simulink model "sim_4_twolink_impedance_control"  (R2021a)
settings: Solver=VariableStepAuto  StartTime=0.0  StopTime=12  MaxStep=0.01  RelTol=1e-3
values from neighbouring files (symbols this model uses):
  b1 = 0.01    [sim_params.m]    (also in sim_params_force.m)
  b2 = 0.01    [sim_params.m]    (also in sim_params_force.m)
  D = [zeros(n); eye(n)]    [control_comparison_script.m]    (also in gen_twolink_ss.m = reshape([0.0,0.0,0.0,0.0,0.0,0.0,0.0,0.0],[4,2]))
  g = 9.80665    [sim_params.m]    (also in sim_params_force.m)
  L1x = 0.3    [sim_params.m]    (also in sim_params_force.m)
  L1y = 0.050    (= 0.05)    [sim_params.m]    (also in sim_params_force.m)
  L1z = 0.05    [sim_params.m]    (also in sim_params_force.m)
  L2x = 0.15    [sim_params.m]    (also in sim_params_force.m = 0.3)
  L2y = 0.05    [sim_params.m]    (also in sim_params_force.m)
  L2z = 0.05    [sim_params.m]    (also in sim_params_force.m)
  m1 = m1*1.25    [control_comparison_script.m]    (also in sim_params.m = 2.775; sim_params_force.m = 2.775)
  m2 = m2*1.25    [control_comparison_script.m]    (also in sim_params.m = 1.3875; sim_params_force.m = 2.775)
  max_joint_torque1 = 20    [sim_params.m]    (also in sim_params_force.m)
  max_joint_torque2 = 10    [sim_params.m]    (also in sim_params_force.m = 20)
  theta1_0 = 0    [sim_params.m]    (also in sim_params_force.m = 1.57079632679)
  theta1_dot_0 = 0    [sim_params.m]    (also in sim_params_force.m)
  theta2_0 = 0    [sim_params.m]    (also in sim_params_force.m = -1.57079632679)
  theta2_dot_0 = 0    [sim_params.m]    (also in sim_params_force.m)
undefined symbols (not defined in the file or in its folder): FT_control, Impedance_no, Kdt, Ke_d, Ke_s, Kpt, Levenberg, Marquardt, Mt_inv, R_env, sigbuilder_block, W_env, X, Xenv, Y, Z
libraries: sm_lib x77, nesl_utility x58, pid_lib x6, simulink x6, robotmaniplib x3, robotcorelib x1
(part 1 of 5)
settings Model: Creator=Petronas-Tareq  LastModifiedBy=Petronas-Tareq
settings ExplorerConfigSet: InternalSimMechanicsExplorerSettings="<ExplorerConfiguration><canonicalview>default</canonicalview><AnimationSetting><BasePlaybackSpeed>1.0</BasePlaybackSpeed><PlaybackSpeedFactor>1.0</PlaybackSpeedFactor></AnimationSetting><TilePanel><TileInfo><Tiles Columns=\"2\" Count=\"4\" Rows=\"2\"><Column Weight=\"0.4998\"/><Column Weight=\"0.5002\"/><Row Weight=\"0.5\"/><Row Weight=\"0.5\"/><Tile Height=\"1\" Width=\"1\" X=\"0\" Y=\"0\"/><Tile Height=\"1\" Width=\"1\" X=\"0\" Y=\"1\"/><Tile Height=\"1\" Width=\"1\" X=\"1\" Y=\"0\"/><Tile Height=\"1\" Width=\"1\" X=\"1\" Y=\"1\"/></Tiles></TileInfo><SceneInfo><SceneViewer><BGColor><R>0.60000002384185791</R><G>0.60000002384185791</G><B>0.60000002384185791</B></BGColor><Camera><DoPerspective>off</DoPerspective><Position><X>0.22866161329300444</X><Y>-0.999999955971509147</Y><Z>-4.12820655437684536e-09</Z></Position><Center><X>0.22866161329300444</X><Y>4.40284908531651742e-08</Y><Z>-4.12820655437684536e-09</Z></Center><Up><X>0</X><Y>-0</Y><Z>1</Z></Up><ViewLimDist>1</ViewLimDist><YLim>0.257500000000000007</YLim><XLim>0.552253577106518345</XLim></Camera></SceneViewer><SceneViewer><BGColor><R>0.60000002384185791</R><G>0.60000002384185791</G><B>0.60000002384185791</B></BGColor><Camera><DoPerspective>off</DoPerspective><Position><X>0.204072367525804987</X><Y>-2.34335064047906805</Y><Z>0.167988192192854713</Z></Position><Center><X>0.219660802383778442</X><Y>-1.34642671678176962</Y><Z>0.0911787457755401237</Z></Center><Up><X>-0.0262288638413234881</X><Y>0.0772000539040926803</Y><Z>0.996670556592697987</Z></Up><ViewLimDist>1</ViewLimDist><YLim>0.515000000000000013</YLim><XLim>1.10450715421303669</XLim></Camera></SceneViewer><SceneViewer><BGColor><R>0.60000002384185791</R><G>0.60000002384185791</G><B>0.60000002384185791</B></BGColor><Camera><DoPerspective>off</DoPerspective><Position><X>-0.24899486320315789</X><Y>-0.765272772333560392</Y><Z>0.697835060620221048</Z></Position><Center><X>0.26973731486207464</X><Y>-0.211131790133127217</Y><Z>0.0468014982858467876</Z></Center><Up><X>0.244353234025975474</X><Y>0.633635300715601257</Y><Z>0.734028475406845016</Z></Up><ViewLimDist>1</ViewLimDist><YLim>0.431008132994174953</YLim><XLim>0.925057201179866673</XLim></Camera></SceneViewer><SceneViewer><BGColor><R>0.60000002384185791</R><G>0.60000002384185791</G><B>0.60000002384185791</B></BGColor><Camera><DoPerspective>off</DoPerspective><Position><X>0.236408339938699752</X><Y>-3.48082895840207129e-09</Y><Z>0.999999999307370047</Z></Position><Center><X>0.236408339938699752</X><Y>-3.48082895840207129e-09</Y><Z>-6.9262995339158806e-10</Z></Center><Up><X>0</X><Y>1</Y><Z>-0</Z></Up><ViewLimDist>1</ViewLimDist><YLim>0.515000000000000013</YLim><XLim>1.10532591414944359</XLim></Camera></SceneViewer></SceneInfo></TilePanel><MechEditorPanel><Cameras/><GfxPanelCameraMap/><VideoCreator><PlaybackSpeedRatio>1.0</PlaybackSpeedRatio><FrameRate>30</FrameRate><VideoFormat>Motion JPEG AVI</VideoFormat><FrameSize>auto</FrameSize></VideoCreator></MechEditorPanel></ExplorerConfiguration>"

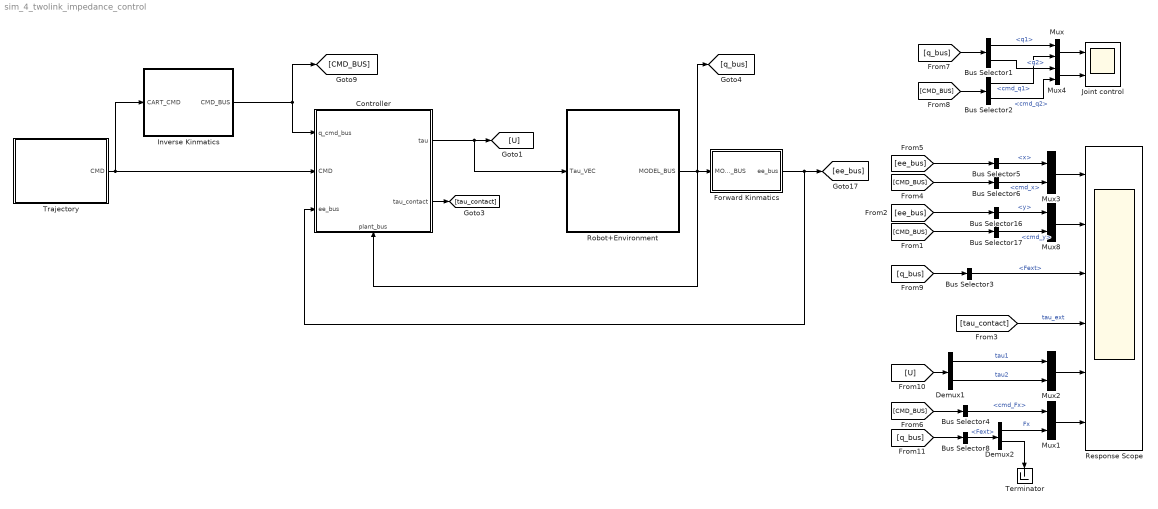
== system sim_4_twolink_impedance_control ==
  Bus Selector1 : BusSelector  OutputSignals=q1,q2
  Bus Selector16 : BusSelector  OutputSignals=y
  Bus Selector17 : BusSelector  OutputSignals=cmd_y
  Bus Selector2 : BusSelector  OutputSignals=cmd_q1,cmd_q2
  Bus Selector3 : BusSelector  OutputSignals=Fext
  Bus Selector4 : BusSelector  OutputSignals=cmd_Fx
  Bus Selector5 : BusSelector  OutputSignals=x
  Bus Selector6 : BusSelector  OutputSignals=cmd_x
  Bus Selector8 : BusSelector  OutputSignals=Fext
  Controller : Subsystem  Variant=on  VariantControlMode=label  LabelModeActiveChoice=Impedance_FT_control  PropagateVariantConditions=on
      settings: PortSchema="{\"entries\":[{\"content\":{\"sides\":[{\"content\":{\"connectorIds\":[\"In1\",\"In2\",\"In3\"]},\"type\":\"ConnectorPlacement.EquallySpacedRectSide\",\"uuid\":\"12e0e0c2-14f8-4f2c-9d40-c223a4f2431c\"},{\"content\":{\"connectorIds\":[\"Out1\",\"Out2\"],\"side\":\"RIGHT\"},\"type\":\"ConnectorPlacement.EquallySpacedRectSide\",\"uuid\":\"b8197539-8519-4525-8d0f-ad401569c0d0\"},{\"content\":{\"connectorIds\":[],\"side\":\"TOP\"},\"type\":\"ConnectorPlacement.EquallySpacedRectSide\",\"uuid\":\"f43dc380-71af-4005-ac59-0dbedf3cc41e\"},{\"content\":{\"connectorIds\":[\"In4\"],\"side\":\"BOTTOM\"},\"type\":\"ConnectorPlacement.EquallySpacedRectSide\",\"uuid\":\"0d04f827-4285-4524-8874-ff3126ed5eeb\"}]},\"type\":\"ConnectorPlacement.EquallySpacedConnector\",\"uuid\":\"aec7d64b-efe7-424b-994a-6b7ee567ecbd\"}],\"packageUris\":[\"http://schema.mathworks.com/mf0/Connector/R2020b\"],\"version\":\"1.0\"}"
  Demux1 : Demux  Outputs=2
  Demux2 : Demux  Outputs=2
  Forward Kinmatics : Subsystem
  Inverse Kinmatics : Subsystem
  Joint control : Scope  NumInputPorts=2
  Mux{,1..4,8} (6 alike) : Mux  Inputs=2
  Response Scope : Scope  NumInputPorts=6
  Robot+Environment : Subsystem  Variant=on  VariantControlMode=label  LabelModeActiveChoice=Choice1
  Terminator : Terminator
  Trajectory : Subsystem  Variant=on  VariantControlMode=label  LabelModeActiveChoice=ramp
  wires:
  Trajectory/1(CMD) -> Inverse Kinmatics/1(CART_CMD), Controller/2(CMD)
  Controller/1(tau) -> [U], Robot+Environment/1(Tau_VEC)
  Robot+Environment/1(MODEL_BUS) -> Controller/4(plant_bus), Forward Kinmatics/1(MODEL_BUS), [q_bus]
  Bus Selector2/1 -> Mux/2  "<cmd_q1>"
  Bus Selector1/2 -> Mux4/1  "<q2>"
  Mux4/1 -> Joint control/2
  [CMD_BUS] -> Bus Selector2/1
  Bus Selector1/1 -> Mux/1  "<q1>"
  Mux/1 -> Joint control/1
  Bus Selector2/2 -> Mux4/2  "<cmd_q2>"
  [q_bus] -> Bus Selector1/1
  Inverse Kinmatics/1(CMD_BUS) -> Controller/1(q_cmd_bus), [CMD_BUS]
  [ee_bus] -> Bus Selector5/1
  [tau_contact] -> Response Scope/4  "tau_ext"
  Bus Selector17/1 -> Mux8/2  "<cmd_y>"
  Mux2/1 -> Response Scope/5
  [U] -> Demux1/1
  [CMD_BUS] -> Bus Selector17/1
  Bus Selector16/1 -> Mux8/1  "<y>"
  Demux1/2 -> Mux2/2  "tau2"
  [ee_bus] -> Bus Selector16/1
  Demux1/1 -> Mux2/1  "tau1"
  Mux8/1 -> Response Scope/2
  Bus Selector6/1 -> Mux3/2  "<cmd_x>"
  [CMD_BUS] -> Bus Selector6/1
  Bus Selector5/1 -> Mux3/1  "<x>"
  Mux3/1 -> Response Scope/1
  Forward Kinmatics/1(ee_bus) -> Controller/3(ee_bus), [ee_bus]
  [q_bus] -> Bus Selector3/1
  Bus Selector3/1 -> Response Scope/3  "<Fext>"
  Controller/2(tau_contact) -> [tau_contact]
  Mux1/1 -> Response Scope/6
  [CMD_BUS] -> Bus Selector4/1
  Bus Selector4/1 -> Mux1/1  "<cmd_Fx>"
  [q_bus] -> Bus Selector8/1
  Bus Selector8/1 -> Demux2/1  "<Fext>"
  Demux2/1 -> Mux1/2  "Fx"
  Demux2/2 -> Terminator/1

== system sim_4_twolink_impedance_control/Controller ==
  note: 1) Add Subsystem or Model blocks as valid variant choices.
      | 2) You cannot connect blocks at this level. At simulation, connectivity is automatically
      | determined, based on the active variant and port name matching.
  q_cmd_bus : Inport
  CMD : Inport  Port=2
  ee_bus : Inport  Port=3
  plant_bus : Inport  Port=4
  "Impedance (with F/T) +Inverse Dynamics control " : Subsystem  VariantControl=Impedance_FT_control
  "Impedance (without F/T) + Inverse Dynamics control " : Subsystem  VariantControl=Impedance_no/FT_control
  Simple complaince Control : Subsystem  VariantControl=simple_complaince_control
  tau : Outport
  tau_contact : Outport  Port=2

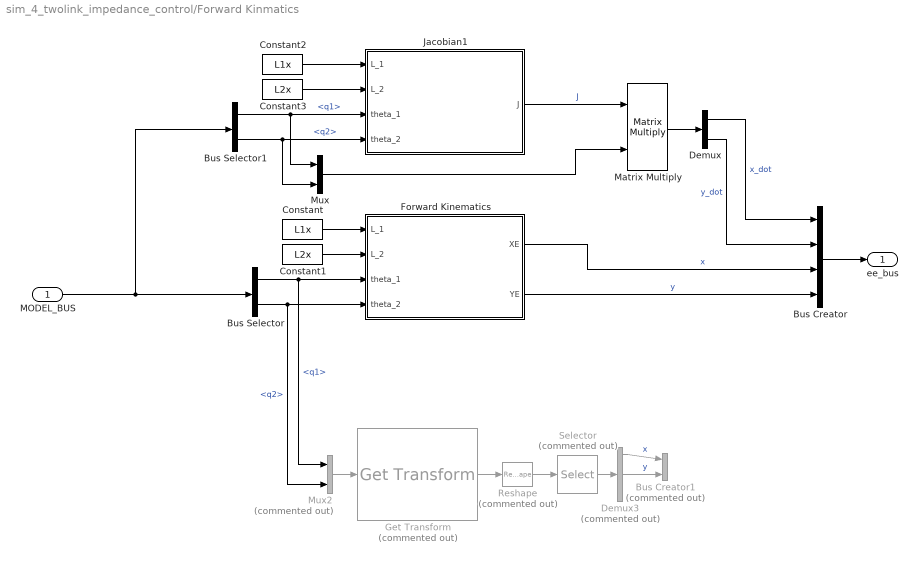
== system sim_4_twolink_impedance_control/Forward Kinmatics ==
  MODEL_BUS : Inport
  Bus Creator : BusCreator  Inputs=4
  Bus Creator1 : BusCreator  Commented=on  Inputs=2
  Bus Selector : BusSelector  OutputSignals=q1,q2
  Bus Selector1 : BusSelector  OutputSignals=q1,q2
  Constant : Constant  Value=L1x
  Constant1 : Constant  Value=L2x
  Constant2 : Constant  Value=L1x
  Constant3 : Constant  Value=L2x
  Demux : Demux  Outputs=2
  Demux3 : Demux  Commented=on  Outputs=3
  Forward Kinematics : MATLAB Function  TreatAsAtomicUnit=on
  Get Transform : robotmaniplib/Get Transform  Commented=on  RigidBodyTree=RR_robot  SourceBody=end_effector  TargetBody=base  SimulateUsing=Interpreted execution
  Jacobian1 : MATLAB Function  TreatAsAtomicUnit=on
  Matrix Multiply : Product  Multiplication=Matrix(*)
  Mux : Mux  Inputs=2
  Mux2 : Mux  Commented=on  Inputs=2
  Reshape : Reshape  Commented=on
  Selector : Selector  Commented=on  InputPortWidth=16  IndexOptions=Index vector (dialog)  Indices=[13:15]  OutputSizes=1
  ee_bus : Outport
  wires:
  Forward Kinematics/2(YE) -> Bus Creator/4  "y"
  Forward Kinematics/1(XE) -> Bus Creator/3  "x"
  Bus Selector/1 -> Mux2/1, Forward Kinematics/3(theta_1)  "<q1>"
  Bus Selector/2 -> Mux2/2, Forward Kinematics/4(theta_2)  "<q2>"
  Constant/1 -> Forward Kinematics/1(L_1)
  Constant1/1 -> Forward Kinematics/2(L_2)
  Mux2/1 -> Get Transform/1
  Get Transform/1 -> Reshape/1
  Reshape/1 -> Selector/1
  Selector/1 -> Demux3/1
  Demux3/1 -> Bus Creator1/1  "x"
  Demux3/2 -> Bus Creator1/2  "y"
  Bus Creator/1 -> ee_bus/1
  Constant2/1 -> Jacobian1/1(L_1)
  Constant3/1 -> Jacobian1/2(L_2)
  Jacobian1/1(J) -> Matrix Multiply/1  "J"
  Bus Selector1/2 -> Mux/2, Jacobian1/4(theta_2)  "<q2>"
  MODEL_BUS/1 -> Bus Selector1/1, Bus Selector/1
  Bus Selector1/1 -> Mux/1, Jacobian1/3(theta_1)  "<q1>"
  Mux/1 -> Matrix Multiply/2
  Matrix Multiply/1 -> Demux/1
  Demux/1 -> Bus Creator/1  "x_dot"
  Demux/2 -> Bus Creator/2  "y_dot"

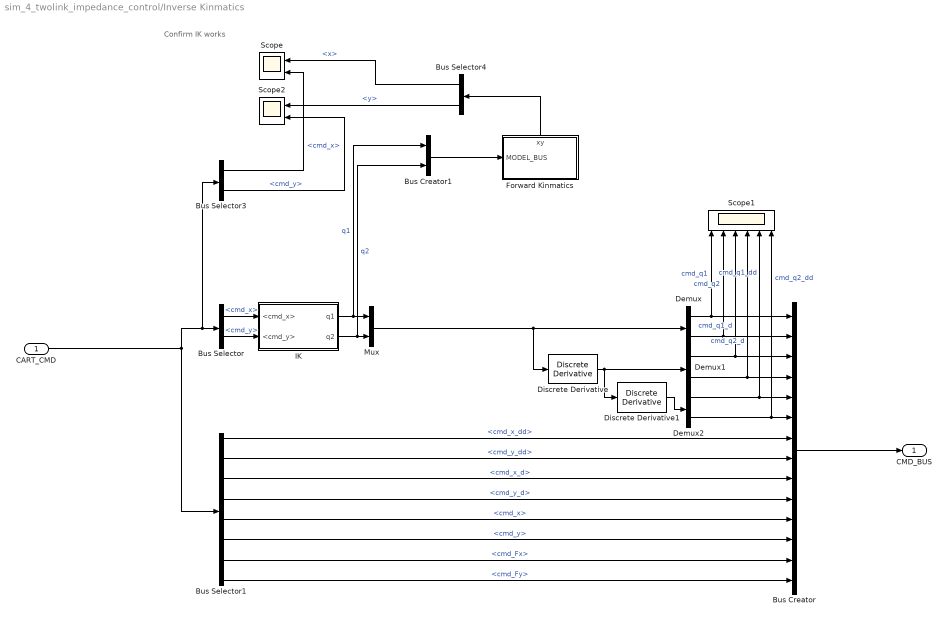
== system sim_4_twolink_impedance_control/Inverse Kinmatics ==
  note: Confirm IK works
  CART_CMD : Inport
  Bus Creator : BusCreator  Inputs=14
  Bus Creator1 : BusCreator  Inputs=2
  Bus Selector : BusSelector  OutputSignals=cmd_x,cmd_y
  Bus Selector1 : BusSelector  OutputSignals=cmd_x_dd,cmd_y_dd,cmd_x_d,cmd_y_d,cmd_x,cmd_y,cmd_Fx,cmd_Fy
  Bus Selector3 : BusSelector  OutputSignals=cmd_x,cmd_y
  Bus Selector4 : BusSelector  OutputSignals=x,y
  Demux : Demux  Outputs=2
  Demux1 : Demux  Outputs=2
  Demux2 : Demux  Outputs=2
  Discrete Derivative : simulink/Discrete/Discrete Derivative  gainval=1.0  ICPrevScaledInput=0.0  OutMin=[]  OutMax=[]  OutDataType=fixdt(1, 16)  OutScaling=2^-10  DoSatur=off
  Discrete Derivative1 : simulink/Discrete/Discrete Derivative  gainval=1.0  ICPrevScaledInput=0.0  OutMin=[]  OutMax=[]  OutDataType=fixdt(1, 16)  OutScaling=2^-10  DoSatur=off
  Forward Kinmatics : Subsystem
      settings: PortSchema="{\"entries\":[{\"content\":{\"sides\":[{\"content\":{\"connectorIds\":[\"In1\"]},\"type\":\"ConnectorPlacement.EquallySpacedRectSide\",\"uuid\":\"2c0f0405-b445-4922-82b0-9ed34ea6e343\"},{\"content\":{\"connectorIds\":[],\"side\":\"RIGHT\"},\"type\":\"ConnectorPlacement.EquallySpacedRectSide\",\"uuid\":\"91fea7c3-4850-470e-b524-5886f9b138cb\"},{\"content\":{\"connectorIds\":[\"Out1\"],\"side\":\"TOP\"},\"type\":\"ConnectorPlacement.EquallySpacedRectSide\",\"uuid\":\"51029b8b-093e-4a55-82a5-f93421c28d2e\"}]},\"type\":\"ConnectorPlacement.EquallySpacedConnector\",\"uuid\":\"843aee16-b8cd-4273-ac03-a5f22ed539be\"}],\"packageUris\":[\"http://schema.mathworks.com/mf0/Connector/R2020b\"],\"version\":\"1.0\"}"
  IK : Subsystem
  Mux : Mux  Inputs=2
  Scope : Scope  NumInputPorts=2
  Scope1 : Scope  NumInputPorts=6
  Scope2 : Scope  NumInputPorts=2
  CMD_BUS : Outport
  wires:
  CART_CMD/1 -> Bus Selector3/1, Bus Selector/1, Bus Selector1/1
  Bus Selector1/1 -> Bus Creator/7  "<cmd_x_dd>"
  Bus Selector1/2 -> Bus Creator/8  "<cmd_y_dd>"
  Bus Selector1/3 -> Bus Creator/9  "<cmd_x_d>"
  Bus Selector1/4 -> Bus Creator/10  "<cmd_y_d>"
  Bus Selector1/5 -> Bus Creator/11  "<cmd_x>"
  Bus Selector1/6 -> Bus Creator/12  "<cmd_y>"
  Demux1/1 -> Scope1/3, Bus Creator/3  "cmd_q1_d"
  Demux2/2 -> Scope1/6, Bus Creator/6  "cmd_q2_dd"
  Demux1/2 -> Scope1/4, Bus Creator/4  "cmd_q2_d"
  Demux/1 -> Scope1/1, Bus Creator/1  "cmd_q1"
  Demux/2 -> Scope1/2, Bus Creator/2  "cmd_q2"
  Bus Selector/1 -> IK/1(<cmd_x>)  "<cmd_x>"
  Bus Selector/2 -> IK/2(<cmd_y>)  "<cmd_y>"
  IK/1(q1) -> Bus Creator1/1, Mux/1  "q1"
  IK/2(q2) -> Bus Creator1/2, Mux/2  "q2"
  Mux/1 -> Demux/1, Discrete Derivative/1
  Discrete Derivative/1 -> Demux1/1, Discrete Derivative1/1
  Demux2/1 -> Scope1/5, Bus Creator/5  "cmd_q1_dd"
  Discrete Derivative1/1 -> Demux2/1
  Bus Creator/1 -> CMD_BUS/1
  Bus Creator1/1 -> Forward Kinmatics/1(MODEL_BUS)
  Forward Kinmatics/1(xy) -> Bus Selector4/1
  Bus Selector3/1 -> Scope/2  "<cmd_x>"
  Bus Selector4/1 -> Scope/1  "<x>"
  Bus Selector4/2 -> Scope2/1  "<y>"
  Bus Selector3/2 -> Scope2/2  "<cmd_y>"
  Bus Selector1/7 -> Bus Creator/13  "<cmd_Fx>"
  Bus Selector1/8 -> Bus Creator/14  "<cmd_Fy>"

== system sim_4_twolink_impedance_control/Robot+Environment ==
  note: 1) Add Subsystem or Model blocks as valid variant choices.
      | 2) You cannot connect blocks at this level. At simulation, connectivity is automatically
      | determined, based on the active variant and port name matching.
  Tau_VEC : Inport
  ARM+Wall Simscape : Subsystem  VariantControl=Choice1
  ARM+Wall Simulink : Subsystem  VariantControl=Choice2
  ARM+curve Simscape : Subsystem  VariantControl=Choice3
  ARM+extrude Simscape : Subsystem  VariantControl=Choice4
  ARM+no constraints Simscape : Subsystem  VariantControl=Choice5
  ARM+ramp up Simscape : Subsystem  VariantControl=Choice6
  MODEL_BUS : Outport

== system sim_4_twolink_impedance_control/Trajectory ==
  note: 1) Add Subsystem or Model blocks as valid variant choices.
      | 2) You cannot connect blocks at this level. At simulation, connectivity is automatically
      | determined, based on the active variant and port name matching.
  Step command : Subsystem  VariantControl=step
  ramp command : Subsystem  VariantControl=ramp
  CMD : Outport

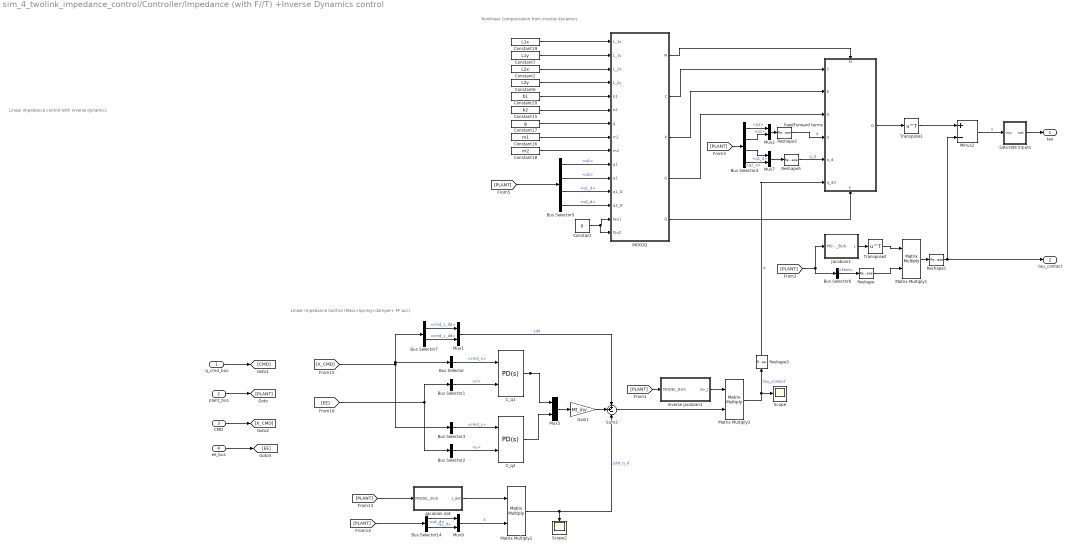
== system sim_4_twolink_impedance_control/Controller/Impedance (with F//T) +Inverse Dynamics control  ==
  note: Linear impedance control with inverse dynamics
  note: Nonlinear Compensation from inverse dynamics
  note: Linear Impedance Control (Mass+Spring+damper+ FF acc)
  q_cmd_bus : Inport
  plant_bus : Inport  Port=2
  CMD : Inport  Port=3
  ee_bus : Inport  Port=4
  Bus Selector : BusSelector  OutputSignals=cmd_x
  Bus Selector1 : BusSelector  OutputSignals=x
  Bus Selector14 : BusSelector  OutputSignals=q1_d,q2_d
  Bus Selector2 : BusSelector  OutputSignals=y
  Bus Selector3 : BusSelector  OutputSignals=cmd_y
  Bus Selector4 : BusSelector  OutputSignals=q1,q2,q1_d,q2_d
  Bus Selector5 : BusSelector  OutputSignals=q1,q2,q1_d,q2_d
  Bus Selector6 : BusSelector  OutputSignals=Fext
  Bus Selector7 : BusSelector  OutputSignals=cmd_x_dd,cmd_y_dd
  C_q1 : pid_lib/PID Controller (2DOF)  Controller=PD  Form=Parallel  TimeDomain=Continuous-time  UseExternalTs=off  SampleTime=-1  IntegratorMethod=Forward Euler  FilterMethod=Forward Euler  ControllerParametersSource=internal  P=Kpt(1)  I=20  D=Kdt(1)  UseFilter=on  N=100  b=1  c=1  TunerSelectOption=Transfer Function Based (PID Tuner App)  InitialConditionSource=internal  InitialConditionForIntegrator=0  InitialConditionForFilter=0  DifferentiatorICPrevScaledInput=0  ExternalReset=none  TrackingMode=off  Kt=1  LimitOutput=off  SatLimitsSource=internal  UpperSaturationLimit=max_joint_torque1  LowerSaturationLimit=-max_joint_torque1  LinearizeAsGain=on  AntiWindupMode=none  Kb=1  POutMin=[]  POutMax=[]  IOutMin=[]  IOutMax=[]  DOutMin=[]  DOutMax=[]  NOutMin=[]  NOutMax=[]  bOutMin=[]  bOutMax=[]  cOutMin=[]  cOutMax=[]  SumOutMin=[]  SumOutMax=[]  SaturationOutMin=[]  SaturationOutMax=[]  PParamMin=[]  PParamMax=[]  IParamMin=[]  IParamMax=[]  DParamMin=[]  DParamMax=[]  NParamMin=[]  NParamMax=[]  bParamMin=[]  bParamMax=[]  cParamMin=[]  cParamMax=[]  KbParamMin=[]  KbParamMax=[]  KtParamMin=[]  KtParamMax=[]  KbOutMin=[]  KbOutMax=[]  KtOutMin=[]  KtOutMax=[]  IntegratorOutMin=[]  IntegratorOutMax=[]  FilterOutMin=[]  FilterOutMax=[]  SumI1OutMin=[]  SumI1OutMax=[]  SumI2OutMin=[]  SumI2OutMax=[]  SumI3OutMin=[]  SumI3OutMax=[]  SumI4OutMin=[]  SumI4OutMax=[]  SumDOutMin=[]  SumDOutMax=[]  Sum1OutMin=[]  Sum1OutMax=[]  Sum2OutMin=[]  Sum2OutMax=[]  Sum3OutMin=[]  Sum3OutMax=[]  DifferentiatorOutMin=[]  DifferentiatorOutMax=[]  FilterDiffOutCoefMin=[]  FilterDiffOutCoefMax=[]  ReciprocalOutMin=[]  ReciprocalOutMax=[]  SumDenOutMin=[]  SumDenOutMax=[]  SumNumOutMin=[]  SumNumOutMax=[]  DivideOutMin=[]  DivideOutMax=[]  UdiffTsProdOutMin=[]  UdiffTsProdOutMax=[]  NTsProdOutMin=[]  NTsProdOutMax=[]  UintegralTsProdOutMin=[]  UintegralTsProdOutMax=[]  UngainTsProdOutMin=[]  UngainTsProdOutMax=[]  IntegratorContinuousStateAttributes=''  IntegratorStateMustResolveToSignalObject=off  IntegratorRTWStateStorageClass=Auto  FilterContinuousStateAttributes=''  FilterStateMustResolveToSignalObject=off  FilterRTWStateStorageClass=Auto  ParallelPVariant=InternalParameters  IdealPVariant=Disabled  IVariant=Disabled  DVariant=InternalParameters  bVariant=InternalParameters  cVariant=InternalParameters  IntegratorVariant=Disabled  SatVariant=Disabled  AWVariant=Disabled  PCopyVariant=Disabled  TRVariant=Disabled  FdbkBlocksVariant=Forward  IdealPFdbkVariant=Disabled  SatFdbkVariant=Disabled  DerivativeFilterVariant=ContFilter  NVariant=InternalParameters  NCopyVariant=Disabled  FilterICVariant=InternalICsFilter  IntegratorICVariant=Disabled  ExternalResetVariant=Disabled  TRSumVariant=Passthrough  SumFdbkVariant=Disabled  SumVariant=Sum_PD  TsampFilterVariant=InternalTs  TsampNgainVariant=Passthrough  TsampIntegralVariant=Disabled_SignalSpec  ExternalSaturationOutDataTypeStr=Inherit: Same as second input
      settings: SourceProductBaseCode=SL
  C_q2 : pid_lib/PID Controller (2DOF)  Controller=PD  Form=Parallel  TimeDomain=Continuous-time  UseExternalTs=off  SampleTime=-1  IntegratorMethod=Forward Euler  FilterMethod=Forward Euler  ControllerParametersSource=internal  P=Kpt(2)  I=20  D=Kdt(2)  UseFilter=on  N=100  b=1  c=1  TunerSelectOption=Transfer Function Based (PID Tuner App)  InitialConditionSource=internal  InitialConditionForIntegrator=0  InitialConditionForFilter=0  DifferentiatorICPrevScaledInput=0  ExternalReset=none  TrackingMode=off  Kt=1  LimitOutput=off  SatLimitsSource=internal  UpperSaturationLimit=max_joint_torque2  LowerSaturationLimit=-max_joint_torque2  LinearizeAsGain=on  AntiWindupMode=none  Kb=1  POutMin=[]  POutMax=[]  IOutMin=[]  IOutMax=[]  DOutMin=[]  DOutMax=[]  NOutMin=[]  NOutMax=[]  bOutMin=[]  bOutMax=[]  cOutMin=[]  cOutMax=[]  SumOutMin=[]  SumOutMax=[]  SaturationOutMin=[]  SaturationOutMax=[]  PParamMin=[]  PParamMax=[]  IParamMin=[]  IParamMax=[]  DParamMin=[]  DParamMax=[]  NParamMin=[]  NParamMax=[]  bParamMin=[]  bParamMax=[]  cParamMin=[]  cParamMax=[]  KbParamMin=[]  KbParamMax=[]  KtParamMin=[]  KtParamMax=[]  KbOutMin=[]  KbOutMax=[]  KtOutMin=[]  KtOutMax=[]  IntegratorOutMin=[]  IntegratorOutMax=[]  FilterOutMin=[]  FilterOutMax=[]  SumI1OutMin=[]  SumI1OutMax=[]  SumI2OutMin=[]  SumI2OutMax=[]  SumI3OutMin=[]  SumI3OutMax=[]  SumI4OutMin=[]  SumI4OutMax=[]  SumDOutMin=[]  SumDOutMax=[]  Sum1OutMin=[]  Sum1OutMax=[]  Sum2OutMin=[]  Sum2OutMax=[]  Sum3OutMin=[]  Sum3OutMax=[]  DifferentiatorOutMin=[]  DifferentiatorOutMax=[]  FilterDiffOutCoefMin=[]  FilterDiffOutCoefMax=[]  ReciprocalOutMin=[]  ReciprocalOutMax=[]  SumDenOutMin=[]  SumDenOutMax=[]  SumNumOutMin=[]  SumNumOutMax=[]  DivideOutMin=[]  DivideOutMax=[]  UdiffTsProdOutMin=[]  UdiffTsProdOutMax=[]  NTsProdOutMin=[]  NTsProdOutMax=[]  UintegralTsProdOutMin=[]  UintegralTsProdOutMax=[]  UngainTsProdOutMin=[]  UngainTsProdOutMax=[]  IntegratorContinuousStateAttributes=''  IntegratorStateMustResolveToSignalObject=off  IntegratorRTWStateStorageClass=Auto  FilterContinuousStateAttributes=''  FilterStateMustResolveToSignalObject=off  FilterRTWStateStorageClass=Auto  ParallelPVariant=InternalParameters  IdealPVariant=Disabled  IVariant=Disabled  DVariant=InternalParameters  bVariant=InternalParameters  cVariant=InternalParameters  IntegratorVariant=Disabled  SatVariant=Disabled  AWVariant=Disabled  PCopyVariant=Disabled  TRVariant=Disabled  FdbkBlocksVariant=Forward  IdealPFdbkVariant=Disabled  SatFdbkVariant=Disabled  DerivativeFilterVariant=ContFilter  NVariant=InternalParameters  NCopyVariant=Disabled  FilterICVariant=InternalICsFilter  IntegratorICVariant=Disabled  ExternalResetVariant=Disabled  TRSumVariant=Passthrough  SumFdbkVariant=Disabled  SumVariant=Sum_PD  TsampFilterVariant=InternalTs  TsampNgainVariant=Passthrough  TsampIntegralVariant=Disabled_SignalSpec  ExternalSaturationOutDataTypeStr=Inherit: Same as second input
      settings: SourceProductBaseCode=SL
  Constant : Constant  Value=0
  Constant15 : Constant  Value=b2
  Constant16 : Constant  Value=m1
  Constant17 : Constant  Value=g
  Constant18 : Constant  Value=m2
  Constant19 : Constant  Value=L1x
  Constant2 : Constant  Value=L2x
  Constant20 : Constant  Value=b1
  Constant6 : Constant  Value=L2y
  Constant7 : Constant  Value=L1y
  FeedForward terms : Subsystem
      settings: PortSchema="{\"entries\":[{\"content\":{\"sides\":[{\"content\":{\"connectorIds\":[\"In1\",\"In2\",\"In3\",\"In4\",\"In5\",\"In6\"]},\"type\":\"ConnectorPlacement.EquallySpacedRectSide\",\"uuid\":\"236e7a2f-027c-4887-b3e9-bc0e11a59ec6\"},{\"content\":{\"connectorIds\":[\"Out1\"],\"side\":\"RIGHT\"},\"type\":\"ConnectorPlacement.EquallySpacedRectSide\",\"uuid\":\"0b727d96-7650-4ea0-95ac-5fb1bad7af10\"},{\"content\":{\"connectorIds\":[\"In7\"],\"side\":\"TOP\"},\"type\":\"ConnectorPlacement.EquallySpacedRectSide\",\"uuid\":\"19d9c8c6-ae7e-49b4-b718-472bd3040569\"},{\"content\":{\"connectorIds\":[\"In8\"],\"side\":\"BOTTOM\"},\"type\":\"ConnectorPlacement.EquallySpacedRectSide\",\"uuid\":\"734f5953-872d-4718-8798-69ea98da43e1\"}]},\"type\":\"ConnectorPlacement.EquallySpacedConnector\",\"uuid\":\"f4b93fea-e2dd-47f1-bf2a-cf2dec03adb9\"}],\"packageUris\":[\"http://schema.mathworks.com/mf0/Connector/R2020b\"],\"version\":\"1.0\"}"
  Gain1 : Gain  Gain=Mt_inv
  Jacobian dot : Subsystem
  Jacobian1 : Subsystem
  MCKGQ : MATLAB Function  TreatAsAtomicUnit=on
  Matrix Multiply1 : Product  Multiplication=Matrix(*)
  Matrix Multiply2 : Product  Multiplication=Matrix(*)
  Matrix Multiply3 : Product  Multiplication=Matrix(*)
  Minus2 : Sum  Inputs=+-
  Mux{1..2,5,7,9} (5 alike) : Mux  Inputs=2
  Reshape{,2..3,5} (4 alike) : Reshape  OutputDimensionality=Column vector (2-D)
  Reshape1 : Reshape  OutputDimensionality=Row vector (2-D)
  Saturate Inputs : Subsystem
  Scope : Scope
  Scope2 : Scope
  Sum2 : Sum  Inputs=++-
  Transpose1 : Math  Operator=transpose  SaturateOnIntegerOverflow=on
  Transpose2 : Math  Operator=transpose  SaturateOnIntegerOverflow=on
  inverse jacobian1 : Subsystem
  tau : Outport
  tau_contact : Outport  Port=2
  wires:
  C_q1/1 -> Mux5/1
  q_cmd_bus/1 -> [CMD]
  plant_bus/1 -> [PLANT]
  Bus Selector2/1 -> C_q2/2  "<y>"
  Bus Selector3/1 -> C_q2/1  "<cmd_y>"
  Bus Selector1/1 -> C_q1/2  "<x>"
  Bus Selector/1 -> C_q1/1  "<cmd_x>"
  [EE] -> Bus Selector1/1, Bus Selector2/1
  Bus Selector5/4 -> MCKGQ/13(q2_D)  "<q2_d>"
  Bus Selector5/3 -> MCKGQ/12(q1_D)  "<q1_d>"
  Bus Selector5/1 -> MCKGQ/10(q1)  "<q1>"
  [PLANT] -> Bus Selector5/1
  Bus Selector5/2 -> MCKGQ/11(q2)  "<q2>"
  FeedForward terms/1(Q) -> Transpose1/1
  [X_CMD] -> Bus Selector7/1, Bus Selector/1, Bus Selector3/1
  C_q2/1 -> Mux5/2
  [PLANT] -> Bus Selector4/1
  Bus Selector4/3 -> Mux7/1  "<q1_d>"
  Bus Selector4/4 -> Mux7/2  "<q2_d>"
  Mux7/1 -> Reshape5/1
  Reshape5/1 -> FeedForward terms/5(q_d)  "q_d"
  MCKGQ/2(C) -> FeedForward terms/1(C)
  MCKGQ/3(K) -> FeedForward terms/2(K)
  MCKGQ/4(G) -> FeedForward terms/3(G)
  Bus Selector4/1 -> Mux2/1  "<q1>"
  Bus Selector4/2 -> Mux2/2  "<q2>"
  Mux2/1 -> Reshape2/1
  Reshape2/1 -> FeedForward terms/4(q)  "q"
  MCKGQ/5(Q) -> FeedForward terms/8(F)
  Constant/1 -> MCKGQ/14(tau1), MCKGQ/15(tau2)
  MCKGQ/1(M) -> FeedForward terms/7(M)
  Constant7/1 -> MCKGQ/2(L_1y)
  Constant2/1 -> MCKGQ/3(L_2x)
  Constant6/1 -> MCKGQ/4(L_2y)
  Constant20/1 -> MCKGQ/5(b1)
  Constant15/1 -> MCKGQ/6(b2)
  Constant17/1 -> MCKGQ/7(g)
  Constant16/1 -> MCKGQ/8(m1)
  Constant18/1 -> MCKGQ/9(m2)
  Constant19/1 -> MCKGQ/1(L_1x)
  Minus2/1 -> Saturate Inputs/1(inp)  "u"
  Matrix Multiply1/1 -> Reshape1/1
  CMD/1 -> [X_CMD]
  ee_bus/1 -> [EE]
  Saturate Inputs/1(sat) -> tau/1
  Transpose1/1 -> Minus2/1
  Matrix Multiply2/1 -> Sum2/3, Scope2/1  "Jdot_q_d"
  Bus Selector14/2 -> Mux9/2  "<q2_d>"
  Bus Selector14/1 -> Mux9/1  "<q1_d>"
  [PLANT] -> Bus Selector14/1
  Mux9/1 -> Matrix Multiply2/2  "X"
  [PLANT] -> Jacobian dot/1(MODEL_BUS)
  Jacobian dot/1(J_dot) -> Matrix Multiply2/1
  [PLANT] -> inverse jacobian1/1(MODEL_BUS)
  Matrix Multiply3/1 -> Reshape3/1, Scope/1  "tau_contact"
  Bus Selector7/1 -> Mux1/1  "<cmd_x_dd>"
  Bus Selector7/2 -> Mux1/2  "<cmd_y_dd>"
  Mux1/1 -> Sum2/1  "xdd"
  Sum2/1 -> Matrix Multiply3/2
  Mux5/1 -> Gain1/1
  Gain1/1 -> Sum2/2
  Reshape3/1 -> FeedForward terms/6(q_dd)  "a"
  inverse jacobian1/1(inv_J) -> Matrix Multiply3/1
  Reshape/1 -> Matrix Multiply1/2
  Bus Selector6/1 -> Reshape/1  "<Fext>"
  [PLANT] -> Bus Selector6/1, Jacobian1/1(MODEL_BUS)
  Jacobian1/1(J) -> Transpose2/1
  Transpose2/1 -> Matrix Multiply1/1
  Reshape1/1 -> tau_contact/1, Minus2/2

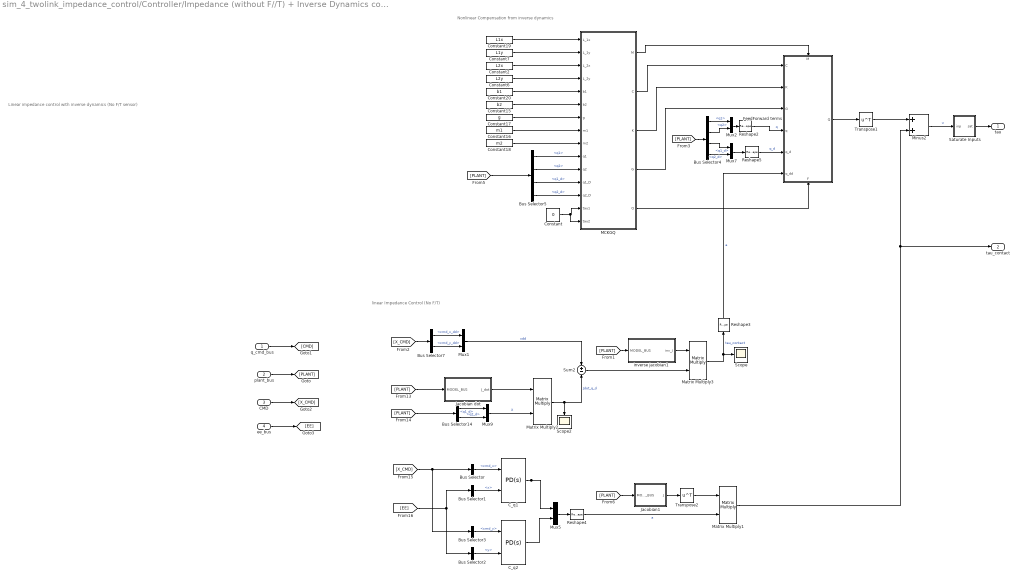
== system sim_4_twolink_impedance_control/Controller/Impedance (without F//T) + Inverse Dynamics control  ==
  note: Linear impedance control with inverse dynamics (No F/T sensor)
  note: Nonlinear Compensation from inverse dynamics
  note: linear Impedance Control (No F/T)
  q_cmd_bus : Inport
  plant_bus : Inport  Port=2
  CMD : Inport  Port=3
  ee_bus : Inport  Port=4
  Bus Selector : BusSelector  OutputSignals=cmd_x
  Bus Selector1 : BusSelector  OutputSignals=x
  Bus Selector14 : BusSelector  OutputSignals=q1_d,q2_d
  Bus Selector2 : BusSelector  OutputSignals=y
  Bus Selector3 : BusSelector  OutputSignals=cmd_y
  Bus Selector4 : BusSelector  OutputSignals=q1,q2,q1_d,q2_d
  Bus Selector5 : BusSelector  OutputSignals=q1,q2,q1_d,q2_d
  Bus Selector7 : BusSelector  OutputSignals=cmd_x_dd,cmd_y_dd
  C_q1 : pid_lib/PID Controller (2DOF)  Controller=PD  Form=Parallel  TimeDomain=Continuous-time  UseExternalTs=off  SampleTime=-1  IntegratorMethod=Forward Euler  FilterMethod=Forward Euler  ControllerParametersSource=internal  P=Kpt(1)  I=20  D=Kdt(1)  UseFilter=on  N=100  b=1  c=1  TunerSelectOption=Transfer Function Based (PID Tuner App)  InitialConditionSource=internal  InitialConditionForIntegrator=0  InitialConditionForFilter=0  DifferentiatorICPrevScaledInput=0  ExternalReset=none  TrackingMode=off  Kt=1  LimitOutput=off  SatLimitsSource=internal  UpperSaturationLimit=max_joint_torque1  LowerSaturationLimit=-max_joint_torque1  LinearizeAsGain=on  AntiWindupMode=none  Kb=1  POutMin=[]  POutMax=[]  IOutMin=[]  IOutMax=[]  DOutMin=[]  DOutMax=[]  NOutMin=[]  NOutMax=[]  bOutMin=[]  bOutMax=[]  cOutMin=[]  cOutMax=[]  SumOutMin=[]  SumOutMax=[]  SaturationOutMin=[]  SaturationOutMax=[]  PParamMin=[]  PParamMax=[]  IParamMin=[]  IParamMax=[]  DParamMin=[]  DParamMax=[]  NParamMin=[]  NParamMax=[]  bParamMin=[]  bParamMax=[]  cParamMin=[]  cParamMax=[]  KbParamMin=[]  KbParamMax=[]  KtParamMin=[]  KtParamMax=[]  KbOutMin=[]  KbOutMax=[]  KtOutMin=[]  KtOutMax=[]  IntegratorOutMin=[]  IntegratorOutMax=[]  FilterOutMin=[]  FilterOutMax=[]  SumI1OutMin=[]  SumI1OutMax=[]  SumI2OutMin=[]  SumI2OutMax=[]  SumI3OutMin=[]  SumI3OutMax=[]  SumI4OutMin=[]  SumI4OutMax=[]  SumDOutMin=[]  SumDOutMax=[]  Sum1OutMin=[]  Sum1OutMax=[]  Sum2OutMin=[]  Sum2OutMax=[]  Sum3OutMin=[]  Sum3OutMax=[]  DifferentiatorOutMin=[]  DifferentiatorOutMax=[]  FilterDiffOutCoefMin=[]  FilterDiffOutCoefMax=[]  ReciprocalOutMin=[]  ReciprocalOutMax=[]  SumDenOutMin=[]  SumDenOutMax=[]  SumNumOutMin=[]  SumNumOutMax=[]  DivideOutMin=[]  DivideOutMax=[]  UdiffTsProdOutMin=[]  UdiffTsProdOutMax=[]  NTsProdOutMin=[]  NTsProdOutMax=[]  UintegralTsProdOutMin=[]  UintegralTsProdOutMax=[]  UngainTsProdOutMin=[]  UngainTsProdOutMax=[]  IntegratorContinuousStateAttributes=''  IntegratorStateMustResolveToSignalObject=off  IntegratorRTWStateStorageClass=Auto  FilterContinuousStateAttributes=''  FilterStateMustResolveToSignalObject=off  FilterRTWStateStorageClass=Auto  ParallelPVariant=InternalParameters  IdealPVariant=Disabled  IVariant=Disabled  DVariant=InternalParameters  bVariant=InternalParameters  cVariant=InternalParameters  IntegratorVariant=Disabled  SatVariant=Disabled  AWVariant=Disabled  PCopyVariant=Disabled  TRVariant=Disabled  FdbkBlocksVariant=Forward  IdealPFdbkVariant=Disabled  SatFdbkVariant=Disabled  DerivativeFilterVariant=ContFilter  NVariant=InternalParameters  NCopyVariant=Disabled  FilterICVariant=InternalICsFilter  IntegratorICVariant=Disabled  ExternalResetVariant=Disabled  TRSumVariant=Passthrough  SumFdbkVariant=Disabled  SumVariant=Sum_PD  TsampFilterVariant=InternalTs  TsampNgainVariant=Passthrough  TsampIntegralVariant=Disabled_SignalSpec  ExternalSaturationOutDataTypeStr=Inherit: Same as second input
      settings: SourceProductBaseCode=SL
  C_q2 : pid_lib/PID Controller (2DOF)  Controller=PD  Form=Parallel  TimeDomain=Continuous-time  UseExternalTs=off  SampleTime=-1  IntegratorMethod=Forward Euler  FilterMethod=Forward Euler  ControllerParametersSource=internal  P=Kpt(2)  I=20  D=Kdt(2)  UseFilter=on  N=100  b=1  c=1  TunerSelectOption=Transfer Function Based (PID Tuner App)  InitialConditionSource=internal  InitialConditionForIntegrator=0  InitialConditionForFilter=0  DifferentiatorICPrevScaledInput=0  ExternalReset=none  TrackingMode=off  Kt=1  LimitOutput=off  SatLimitsSource=internal  UpperSaturationLimit=max_joint_torque2  LowerSaturationLimit=-max_joint_torque2  LinearizeAsGain=on  AntiWindupMode=none  Kb=1  POutMin=[]  POutMax=[]  IOutMin=[]  IOutMax=[]  DOutMin=[]  DOutMax=[]  NOutMin=[]  NOutMax=[]  bOutMin=[]  bOutMax=[]  cOutMin=[]  cOutMax=[]  SumOutMin=[]  SumOutMax=[]  SaturationOutMin=[]  SaturationOutMax=[]  PParamMin=[]  PParamMax=[]  IParamMin=[]  IParamMax=[]  DParamMin=[]  DParamMax=[]  NParamMin=[]  NParamMax=[]  bParamMin=[]  bParamMax=[]  cParamMin=[]  cParamMax=[]  KbParamMin=[]  KbParamMax=[]  KtParamMin=[]  KtParamMax=[]  KbOutMin=[]  KbOutMax=[]  KtOutMin=[]  KtOutMax=[]  IntegratorOutMin=[]  IntegratorOutMax=[]  FilterOutMin=[]  FilterOutMax=[]  SumI1OutMin=[]  SumI1OutMax=[]  SumI2OutMin=[]  SumI2OutMax=[]  SumI3OutMin=[]  SumI3OutMax=[]  SumI4OutMin=[]  SumI4OutMax=[]  SumDOutMin=[]  SumDOutMax=[]  Sum1OutMin=[]  Sum1OutMax=[]  Sum2OutMin=[]  Sum2OutMax=[]  Sum3OutMin=[]  Sum3OutMax=[]  DifferentiatorOutMin=[]  DifferentiatorOutMax=[]  FilterDiffOutCoefMin=[]  FilterDiffOutCoefMax=[]  ReciprocalOutMin=[]  ReciprocalOutMax=[]  SumDenOutMin=[]  SumDenOutMax=[]  SumNumOutMin=[]  SumNumOutMax=[]  DivideOutMin=[]  DivideOutMax=[]  UdiffTsProdOutMin=[]  UdiffTsProdOutMax=[]  NTsProdOutMin=[]  NTsProdOutMax=[]  UintegralTsProdOutMin=[]  UintegralTsProdOutMax=[]  UngainTsProdOutMin=[]  UngainTsProdOutMax=[]  IntegratorContinuousStateAttributes=''  IntegratorStateMustResolveToSignalObject=off  IntegratorRTWStateStorageClass=Auto  FilterContinuousStateAttributes=''  FilterStateMustResolveToSignalObject=off  FilterRTWStateStorageClass=Auto  ParallelPVariant=InternalParameters  IdealPVariant=Disabled  IVariant=Disabled  DVariant=InternalParameters  bVariant=InternalParameters  cVariant=InternalParameters  IntegratorVariant=Disabled  SatVariant=Disabled  AWVariant=Disabled  PCopyVariant=Disabled  TRVariant=Disabled  FdbkBlocksVariant=Forward  IdealPFdbkVariant=Disabled  SatFdbkVariant=Disabled  DerivativeFilterVariant=ContFilter  NVariant=InternalParameters  NCopyVariant=Disabled  FilterICVariant=InternalICsFilter  IntegratorICVariant=Disabled  ExternalResetVariant=Disabled  TRSumVariant=Passthrough  SumFdbkVariant=Disabled  SumVariant=Sum_PD  TsampFilterVariant=InternalTs  TsampNgainVariant=Passthrough  TsampIntegralVariant=Disabled_SignalSpec  ExternalSaturationOutDataTypeStr=Inherit: Same as second input
      settings: SourceProductBaseCode=SL
  Constant : Constant  Value=0
  Constant15 : Constant  Value=b2
  Constant16 : Constant  Value=m1
  Constant17 : Constant  Value=g
  Constant18 : Constant  Value=m2
  Constant19 : Constant  Value=L1x
  Constant2 : Constant  Value=L2x
  Constant20 : Constant  Value=b1
  Constant6 : Constant  Value=L2y
  Constant7 : Constant  Value=L1y
  FeedForward terms : Subsystem
      settings: PortSchema="{\"entries\":[{\"content\":{\"sides\":[{\"content\":{\"connectorIds\":[\"In1\",\"In2\",\"In3\",\"In4\",\"In5\",\"In6\"]},\"type\":\"ConnectorPlacement.EquallySpacedRectSide\",\"uuid\":\"236e7a2f-027c-4887-b3e9-bc0e11a59ec6\"},{\"content\":{\"connectorIds\":[\"Out1\"],\"side\":\"RIGHT\"},\"type\":\"ConnectorPlacement.EquallySpacedRectSide\",\"uuid\":\"0b727d96-7650-4ea0-95ac-5fb1bad7af10\"},{\"content\":{\"connectorIds\":[\"In7\"],\"side\":\"TOP\"},\"type\":\"ConnectorPlacement.EquallySpacedRectSide\",\"uuid\":\"19d9c8c6-ae7e-49b4-b718-472bd3040569\"},{\"content\":{\"connectorIds\":[\"In8\"],\"side\":\"BOTTOM\"},\"type\":\"ConnectorPlacement.EquallySpacedRectSide\",\"uuid\":\"734f5953-872d-4718-8798-69ea98da43e1\"}]},\"type\":\"ConnectorPlacement.EquallySpacedConnector\",\"uuid\":\"f4b93fea-e2dd-47f1-bf2a-cf2dec03adb9\"}],\"packageUris\":[\"http://schema.mathworks.com/mf0/Connector/R2020b\"],\"version\":\"1.0\"}"
  Jacobian dot : Subsystem
  Jacobian1 : Subsystem
  MCKGQ : MATLAB Function  TreatAsAtomicUnit=on
  Matrix Multiply1 : Product  Multiplication=Matrix(*)
  Matrix Multiply2 : Product  Multiplication=Matrix(*)
  Matrix Multiply3 : Product  Multiplication=Matrix(*)
  Minus2 : Sum
  Mux{1..2,5,7,9} (5 alike) : Mux  Inputs=2
  Reshape2 : Reshape  OutputDimensionality=Column vector (2-D)
  Reshape3 : Reshape  OutputDimensionality=Column vector (2-D)
  Reshape4 : Reshape  OutputDimensionality=Row vector (2-D)
  Reshape5 : Reshape  OutputDimensionality=Column vector (2-D)
  Saturate Inputs : Subsystem
  Scope : Scope
  Scope2 : Scope
  Sum2 : Sum  Inputs=+|-
  Transpose1 : Math  Operator=transpose  SaturateOnIntegerOverflow=on
  Transpose2 : Math  Operator=transpose  SaturateOnIntegerOverflow=on
  inverse jacobian1 : Subsystem
  tau : Outport
  tau_contact : Outport  Port=2
  wires:
  q_cmd_bus/1 -> [CMD]
  plant_bus/1 -> [PLANT]
  Bus Selector5/4 -> MCKGQ/13(q2_D)  "<q2_d>"
  Bus Selector5/3 -> MCKGQ/12(q1_D)  "<q1_d>"
  Bus Selector5/1 -> MCKGQ/10(q1)  "<q1>"
  [PLANT] -> Bus Selector5/1
  Bus Selector5/2 -> MCKGQ/11(q2)  "<q2>"
  FeedForward terms/1(Q) -> Transpose1/1
  [PLANT] -> Bus Selector4/1
  Bus Selector4/3 -> Mux7/1  "<q1_d>"
  Bus Selector4/4 -> Mux7/2  "<q2_d>"
  Mux7/1 -> Reshape5/1
  Reshape5/1 -> FeedForward terms/5(q_d)  "q_d"
  MCKGQ/2(C) -> FeedForward terms/1(C)
  MCKGQ/3(K) -> FeedForward terms/2(K)
  MCKGQ/4(G) -> FeedForward terms/3(G)
  Bus Selector4/1 -> Mux2/1  "<q1>"
  Bus Selector4/2 -> Mux2/2  "<q2>"
  Mux2/1 -> Reshape2/1
  Reshape2/1 -> FeedForward terms/4(q)  "q"
  MCKGQ/5(Q) -> FeedForward terms/8(F)
  Constant/1 -> MCKGQ/14(tau1), MCKGQ/15(tau2)
  MCKGQ/1(M) -> FeedForward terms/7(M)
  Constant7/1 -> MCKGQ/2(L_1y)
  Constant2/1 -> MCKGQ/3(L_2x)
  Constant6/1 -> MCKGQ/4(L_2y)
  Constant20/1 -> MCKGQ/5(b1)
  Constant15/1 -> MCKGQ/6(b2)
  Constant17/1 -> MCKGQ/7(g)
  Constant16/1 -> MCKGQ/8(m1)
  Constant18/1 -> MCKGQ/9(m2)
  Constant19/1 -> MCKGQ/1(L_1x)
  Minus2/1 -> Saturate Inputs/1(inp)  "u"
  Matrix Multiply1/1 -> tau_contact/1, Minus2/2
  CMD/1 -> [X_CMD]
  ee_bus/1 -> [EE]
  Saturate Inputs/1(sat) -> tau/1
  Transpose1/1 -> Minus2/1
  Matrix Multiply2/1 -> Sum2/2, Scope2/1  "Jdot_q_d"
  Bus Selector14/2 -> Mux9/2  "<q2_d>"
  Bus Selector14/1 -> Mux9/1  "<q1_d>"
  [PLANT] -> Bus Selector14/1
  Mux9/1 -> Matrix Multiply2/2  "X"
  [PLANT] -> Jacobian dot/1(MODEL_BUS)
  Jacobian dot/1(J_dot) -> Matrix Multiply2/1
  [PLANT] -> inverse jacobian1/1(MODEL_BUS)
  Matrix Multiply3/1 -> Reshape3/1, Scope/1  "tau_contact"
  Bus Selector7/1 -> Mux1/1  "<cmd_x_dd>"
  Bus Selector7/2 -> Mux1/2  "<cmd_y_dd>"
  Mux1/1 -> Sum2/1  "xdd"
  Sum2/1 -> Matrix Multiply3/2
  Reshape3/1 -> FeedForward terms/6(q_dd)  "a"
  C_q2/1 -> Mux5/2
  [EE] -> Bus Selector1/1, Bus Selector2/1
  Bus Selector1/1 -> C_q1/2  "<x>"
  [X_CMD] -> Bus Selector3/1, Bus Selector/1
  Bus Selector/1 -> C_q1/1  "<cmd_x>"
  Bus Selector3/1 -> C_q2/1  "<cmd_y>"
  Bus Selector2/1 -> C_q2/2  "<y>"
  C_q1/1 -> Mux5/1
  [X_CMD] -> Bus Selector7/1
  Jacobian1/1(J) -> Transpose2/1
  [PLANT] -> Jacobian1/1(MODEL_BUS)
  Transpose2/1 -> Matrix Multiply1/1
  Mux5/1 -> Reshape4/1
  Reshape4/1 -> Matrix Multiply1/2  "a"
  inverse jacobian1/1(inv_J) -> Matrix Multiply3/1

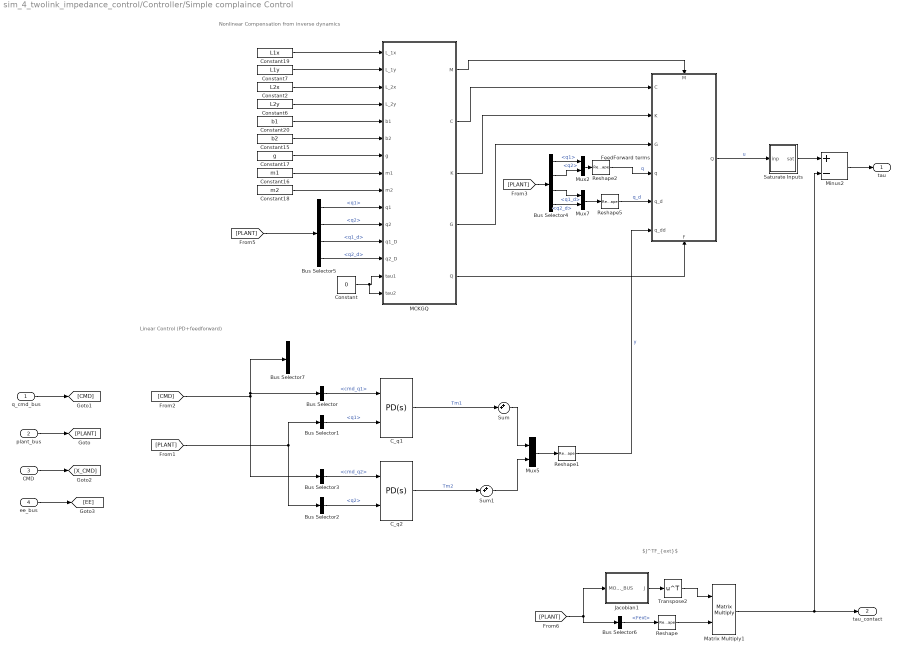
== system sim_4_twolink_impedance_control/Controller/Simple complaince Control ==
  note: $J^TF_{ext}$
  note: Nonlinear Compensation from inverse dynamics
  note: Linear Control (PD+feedforward)
  q_cmd_bus : Inport
  plant_bus : Inport  Port=2
  CMD : Inport  Port=3
  ee_bus : Inport  Port=4
  Bus Selector : BusSelector  OutputSignals=cmd_q1
  Bus Selector1 : BusSelector  OutputSignals=q1
  Bus Selector2 : BusSelector  OutputSignals=q2
  Bus Selector3 : BusSelector  OutputSignals=cmd_q2
  Bus Selector4 : BusSelector  OutputSignals=q1,q2,q1_d,q2_d
  Bus Selector5 : BusSelector  OutputSignals=q1,q2,q1_d,q2_d
  Bus Selector6 : BusSelector  OutputSignals=Fext
  Bus Selector7 : BusSelector  OutputSignals=cmd_q1_dd,cmd_q2_dd
  C_q1 : pid_lib/PID Controller (2DOF)  Controller=PD  Form=Parallel  TimeDomain=Continuous-time  UseExternalTs=off  SampleTime=-1  IntegratorMethod=Forward Euler  FilterMethod=Forward Euler  ControllerParametersSource=internal  P=400  I=20  D=40  UseFilter=on  N=100  b=1  c=1  TunerSelectOption=Transfer Function Based (PID Tuner App)  InitialConditionSource=internal  InitialConditionForIntegrator=0  InitialConditionForFilter=0  DifferentiatorICPrevScaledInput=0  ExternalReset=none  TrackingMode=off  Kt=1  LimitOutput=off  SatLimitsSource=internal  UpperSaturationLimit=max_joint_torque1  LowerSaturationLimit=-max_joint_torque1  LinearizeAsGain=on  AntiWindupMode=none  Kb=1  POutMin=[]  POutMax=[]  IOutMin=[]  IOutMax=[]  DOutMin=[]  DOutMax=[]  NOutMin=[]  NOutMax=[]  bOutMin=[]  bOutMax=[]  cOutMin=[]  cOutMax=[]  SumOutMin=[]  SumOutMax=[]  SaturationOutMin=[]  SaturationOutMax=[]  PParamMin=[]  PParamMax=[]  IParamMin=[]  IParamMax=[]  DParamMin=[]  DParamMax=[]  NParamMin=[]  NParamMax=[]  bParamMin=[]  bParamMax=[]  cParamMin=[]  cParamMax=[]  KbParamMin=[]  KbParamMax=[]  KtParamMin=[]  KtParamMax=[]  KbOutMin=[]  KbOutMax=[]  KtOutMin=[]  KtOutMax=[]  IntegratorOutMin=[]  IntegratorOutMax=[]  FilterOutMin=[]  FilterOutMax=[]  SumI1OutMin=[]  SumI1OutMax=[]  SumI2OutMin=[]  SumI2OutMax=[]  SumI3OutMin=[]  SumI3OutMax=[]  SumI4OutMin=[]  SumI4OutMax=[]  SumDOutMin=[]  SumDOutMax=[]  Sum1OutMin=[]  Sum1OutMax=[]  Sum2OutMin=[]  Sum2OutMax=[]  Sum3OutMin=[]  Sum3OutMax=[]  DifferentiatorOutMin=[]  DifferentiatorOutMax=[]  FilterDiffOutCoefMin=[]  FilterDiffOutCoefMax=[]  ReciprocalOutMin=[]  ReciprocalOutMax=[]  SumDenOutMin=[]  SumDenOutMax=[]  SumNumOutMin=[]  SumNumOutMax=[]  DivideOutMin=[]  DivideOutMax=[]  UdiffTsProdOutMin=[]  UdiffTsProdOutMax=[]  NTsProdOutMin=[]  NTsProdOutMax=[]  UintegralTsProdOutMin=[]  UintegralTsProdOutMax=[]  UngainTsProdOutMin=[]  UngainTsProdOutMax=[]  IntegratorContinuousStateAttributes=''  IntegratorStateMustResolveToSignalObject=off  IntegratorRTWStateStorageClass=Auto  FilterContinuousStateAttributes=''  FilterStateMustResolveToSignalObject=off  FilterRTWStateStorageClass=Auto  ParallelPVariant=InternalParameters  IdealPVariant=Disabled  IVariant=Disabled  DVariant=InternalParameters  bVariant=InternalParameters  cVariant=InternalParameters  IntegratorVariant=Disabled  SatVariant=Disabled  AWVariant=Disabled  PCopyVariant=Disabled  TRVariant=Disabled  FdbkBlocksVariant=Forward  IdealPFdbkVariant=Disabled  SatFdbkVariant=Disabled  DerivativeFilterVariant=ContFilter  NVariant=InternalParameters  NCopyVariant=Disabled  FilterICVariant=InternalICsFilter  IntegratorICVariant=Disabled  ExternalResetVariant=Disabled  TRSumVariant=Passthrough  SumFdbkVariant=Disabled  SumVariant=Sum_PD  TsampFilterVariant=InternalTs  TsampNgainVariant=Passthrough  TsampIntegralVariant=Disabled_SignalSpec  ExternalSaturationOutDataTypeStr=Inherit: Same as second input
      settings: SourceProductBaseCode=SL
  C_q2 : pid_lib/PID Controller (2DOF)  Controller=PD  Form=Parallel  TimeDomain=Continuous-time  UseExternalTs=off  SampleTime=-1  IntegratorMethod=Forward Euler  FilterMethod=Forward Euler  ControllerParametersSource=internal  P=200  I=20  D=35  UseFilter=on  N=100  b=1  c=1  TunerSelectOption=Transfer Function Based (PID Tuner App)  InitialConditionSource=internal  InitialConditionForIntegrator=0  InitialConditionForFilter=0  DifferentiatorICPrevScaledInput=0  ExternalReset=none  TrackingMode=off  Kt=1  LimitOutput=off  SatLimitsSource=internal  UpperSaturationLimit=max_joint_torque2  LowerSaturationLimit=-max_joint_torque2  LinearizeAsGain=on  AntiWindupMode=none  Kb=1  POutMin=[]  POutMax=[]  IOutMin=[]  IOutMax=[]  DOutMin=[]  DOutMax=[]  NOutMin=[]  NOutMax=[]  bOutMin=[]  bOutMax=[]  cOutMin=[]  cOutMax=[]  SumOutMin=[]  SumOutMax=[]  SaturationOutMin=[]  SaturationOutMax=[]  PParamMin=[]  PParamMax=[]  IParamMin=[]  IParamMax=[]  DParamMin=[]  DParamMax=[]  NParamMin=[]  NParamMax=[]  bParamMin=[]  bParamMax=[]  cParamMin=[]  cParamMax=[]  KbParamMin=[]  KbParamMax=[]  KtParamMin=[]  KtParamMax=[]  KbOutMin=[]  KbOutMax=[]  KtOutMin=[]  KtOutMax=[]  IntegratorOutMin=[]  IntegratorOutMax=[]  FilterOutMin=[]  FilterOutMax=[]  SumI1OutMin=[]  SumI1OutMax=[]  SumI2OutMin=[]  SumI2OutMax=[]  SumI3OutMin=[]  SumI3OutMax=[]  SumI4OutMin=[]  SumI4OutMax=[]  SumDOutMin=[]  SumDOutMax=[]  Sum1OutMin=[]  Sum1OutMax=[]  Sum2OutMin=[]  Sum2OutMax=[]  Sum3OutMin=[]  Sum3OutMax=[]  DifferentiatorOutMin=[]  DifferentiatorOutMax=[]  FilterDiffOutCoefMin=[]  FilterDiffOutCoefMax=[]  ReciprocalOutMin=[]  ReciprocalOutMax=[]  SumDenOutMin=[]  SumDenOutMax=[]  SumNumOutMin=[]  SumNumOutMax=[]  DivideOutMin=[]  DivideOutMax=[]  UdiffTsProdOutMin=[]  UdiffTsProdOutMax=[]  NTsProdOutMin=[]  NTsProdOutMax=[]  UintegralTsProdOutMin=[]  UintegralTsProdOutMax=[]  UngainTsProdOutMin=[]  UngainTsProdOutMax=[]  IntegratorContinuousStateAttributes=''  IntegratorStateMustResolveToSignalObject=off  IntegratorRTWStateStorageClass=Auto  FilterContinuousStateAttributes=''  FilterStateMustResolveToSignalObject=off  FilterRTWStateStorageClass=Auto  ParallelPVariant=InternalParameters  IdealPVariant=Disabled  IVariant=Disabled  DVariant=InternalParameters  bVariant=InternalParameters  cVariant=InternalParameters  IntegratorVariant=Disabled  SatVariant=Disabled  AWVariant=Disabled  PCopyVariant=Disabled  TRVariant=Disabled  FdbkBlocksVariant=Forward  IdealPFdbkVariant=Disabled  SatFdbkVariant=Disabled  DerivativeFilterVariant=ContFilter  NVariant=InternalParameters  NCopyVariant=Disabled  FilterICVariant=InternalICsFilter  IntegratorICVariant=Disabled  ExternalResetVariant=Disabled  TRSumVariant=Passthrough  SumFdbkVariant=Disabled  SumVariant=Sum_PD  TsampFilterVariant=InternalTs  TsampNgainVariant=Passthrough  TsampIntegralVariant=Disabled_SignalSpec  ExternalSaturationOutDataTypeStr=Inherit: Same as second input
      settings: SourceProductBaseCode=SL
  Constant : Constant  Value=0
  Constant15 : Constant  Value=b2
  Constant16 : Constant  Value=m1
  Constant17 : Constant  Value=g
  Constant18 : Constant  Value=m2
  Constant19 : Constant  Value=L1x
  Constant2 : Constant  Value=L2x
  Constant20 : Constant  Value=b1
  Constant6 : Constant  Value=L2y
  Constant7 : Constant  Value=L1y
  FeedForward terms : Subsystem
      settings: PortSchema="{\"entries\":[{\"content\":{\"sides\":[{\"content\":{\"connectorIds\":[\"In1\",\"In2\",\"In3\",\"In4\",\"In5\",\"In6\"]},\"type\":\"ConnectorPlacement.EquallySpacedRectSide\",\"uuid\":\"236e7a2f-027c-4887-b3e9-bc0e11a59ec6\"},{\"content\":{\"connectorIds\":[\"Out1\"],\"side\":\"RIGHT\"},\"type\":\"ConnectorPlacement.EquallySpacedRectSide\",\"uuid\":\"0b727d96-7650-4ea0-95ac-5fb1bad7af10\"},{\"content\":{\"connectorIds\":[\"In7\"],\"side\":\"TOP\"},\"type\":\"ConnectorPlacement.EquallySpacedRectSide\",\"uuid\":\"19d9c8c6-ae7e-49b4-b718-472bd3040569\"},{\"content\":{\"connectorIds\":[\"In8\"],\"side\":\"BOTTOM\"},\"type\":\"ConnectorPlacement.EquallySpacedRectSide\",\"uuid\":\"734f5953-872d-4718-8798-69ea98da43e1\"}]},\"type\":\"ConnectorPlacement.EquallySpacedConnector\",\"uuid\":\"f4b93fea-e2dd-47f1-bf2a-cf2dec03adb9\"}],\"packageUris\":[\"http://schema.mathworks.com/mf0/Connector/R2020b\"],\"version\":\"1.0\"}"
  Jacobian1 : Subsystem
  MCKGQ : MATLAB Function  TreatAsAtomicUnit=on
  Matrix Multiply1 : Product  Multiplication=Matrix(*)
  Minus2 : Sum  Inputs=+-
  Mux2 : Mux  Inputs=2
  Mux5 : Mux  Inputs=2
  Mux7 : Mux  Inputs=2
  Reshape{,1..2,5} (4 alike) : Reshape  OutputDimensionality=Column vector (2-D)
  Saturate Inputs : Subsystem
  Sum : Sum  Inputs=++|
  Sum1 : Sum  Inputs=++|
  Transpose2 : Math  Operator=transpose  SaturateOnIntegerOverflow=on
  tau : Outport
  tau_contact : Outport  Port=2
  wires:
  CMD/1 -> [X_CMD]
  Minus2/1 -> tau/1
  Sum1/1 -> Mux5/2
  Constant17/1 -> MCKGQ/7(g)
  Matrix Multiply1/1 -> tau_contact/1, Minus2/2
  MCKGQ/4(G) -> FeedForward terms/3(G)
  Constant7/1 -> MCKGQ/2(L_1y)
  Mux2/1 -> Reshape2/1
  Mux7/1 -> Reshape5/1
  Constant20/1 -> MCKGQ/5(b1)
  Constant19/1 -> MCKGQ/1(L_1x)
  Sum/1 -> Mux5/1
  Constant2/1 -> MCKGQ/3(L_2x)
  Constant15/1 -> MCKGQ/6(b2)
  MCKGQ/3(K) -> FeedForward terms/2(K)
  Reshape1/1 -> FeedForward terms/6(q_dd)  "y"
  MCKGQ/2(C) -> FeedForward terms/1(C)
  MCKGQ/1(M) -> FeedForward terms/7(M)
  Bus Selector4/3 -> Mux7/1  "<q1_d>"
  Bus Selector4/1 -> Mux2/1  "<q1>"
  Reshape2/1 -> FeedForward terms/4(q)  "q"
  Bus Selector/1 -> C_q1/1  "<cmd_q1>"
  C_q2/1 -> Sum1/2  "Tm2"
  plant_bus/1 -> [PLANT]
  q_cmd_bus/1 -> [CMD]
  Bus Selector2/1 -> C_q2/2  "<q2>"
  [PLANT] -> Bus Selector1/1, Bus Selector2/1
  Reshape5/1 -> FeedForward terms/5(q_d)  "q_d"
  FeedForward terms/1(Q) -> Saturate Inputs/1(inp)  "u"
  [PLANT] -> Bus Selector5/1
  Bus Selector5/2 -> MCKGQ/11(q2)  "<q2>"
  Bus Selector4/4 -> Mux7/2  "<q2_d>"
  Bus Selector5/3 -> MCKGQ/12(q1_D)  "<q1_d>"
  [PLANT] -> Bus Selector4/1
  Bus Selector5/4 -> MCKGQ/13(q2_D)  "<q2_d>"
  C_q1/1 -> Sum/2  "Tm1"
  Bus Selector1/1 -> C_q1/2  "<q1>"
  Constant16/1 -> MCKGQ/8(m1)
  MCKGQ/5(Q) -> FeedForward terms/8(F)
  Constant/1 -> MCKGQ/14(tau1), MCKGQ/15(tau2)
  Constant18/1 -> MCKGQ/9(m2)
  ee_bus/1 -> [EE]
  Bus Selector5/1 -> MCKGQ/10(q1)  "<q1>"
  Saturate Inputs/1(sat) -> Minus2/1
  Mux5/1 -> Reshape1/1
  Constant6/1 -> MCKGQ/4(L_2y)
  [CMD] -> Bus Selector7/1, Bus Selector/1, Bus Selector3/1
  Bus Selector3/1 -> C_q2/1  "<cmd_q2>"
  Bus Selector4/2 -> Mux2/2  "<q2>"
  Bus Selector6/1 -> Reshape/1  "<Fext>"
  [PLANT] -> Bus Selector6/1, Jacobian1/1(MODEL_BUS)
  Reshape/1 -> Matrix Multiply1/2
  Jacobian1/1(J) -> Transpose2/1
  Transpose2/1 -> Matrix Multiply1/1
